simulink model "Active_Suspension_System"  (R2025b)
settings: Solver=ode45  StartTime=0.0  StopTime=10.0  RelTol=1e-3
undefined symbols (not defined in the file): cs, ct, Kd, Ki, Kp, ks, kt, ms, mus
libraries: slpidlib x1, simulink x1
settings Model: Creator=manikantagonugondla  LastModifiedBy=manikantagonugondla

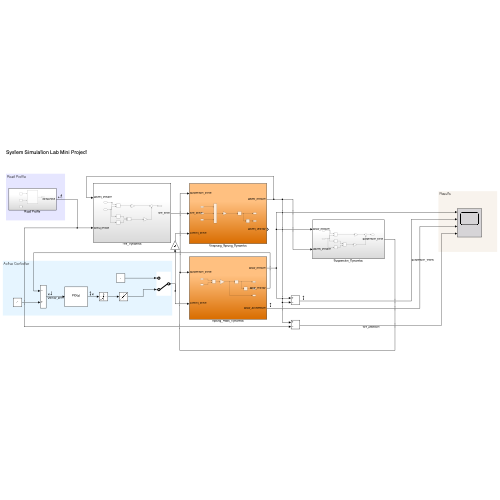
[thumbnail: Simulink's stored preview of the top-level diagram]
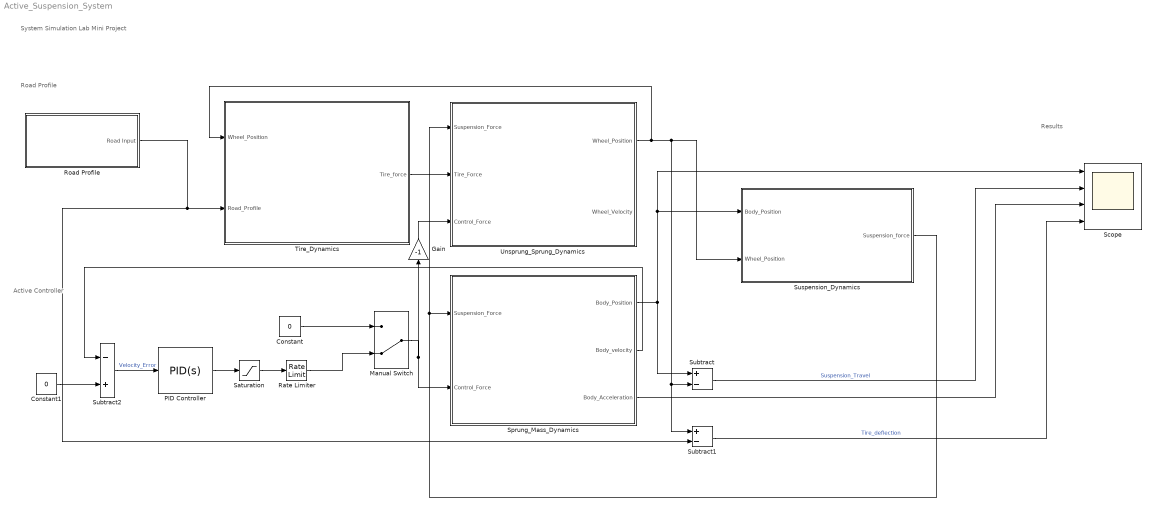
== system Active_Suspension_System ==
  note: Active Controller
  note: System Simulation Lab Mini Project
  note: Results
  note: Road Profile
  Constant : Constant  Value=0
  Constant1 : Constant  Value=0
  Gain : Gain  Gain=-1
  Manual Switch : ManualSwitch  CurrentSetting=0
  PID Controller : slpidlib/PID Controller  Controller=PID  Form=Parallel  TimeDomain=Continuous-time  UseExternalTs=off  SampleTime=-1  IntegratorMethod=Forward Euler  FilterMethod=Forward Euler  ControllerParametersSource=internal  P=Kp  I=Ki  UseKiTs=off  D=Kd  UseExternalDerivativeSource=off  N=50  UseFilter=on  TunerSelectOption=Transfer Function Based (PID Tuner App)  InitialConditionSource=internal  InitialConditionForIntegrator=0  InitialConditionForFilter=0  DifferentiatorICPrevScaledInput=0  ExternalReset=none  TrackingMode=off  Kt=1  LimitOutput=off  SatLimitsSource=internal  UpperSaturationLimit=inf  LowerSaturationLimit=-inf  LinearizeAsGain=on  AntiWindupMode=none  Kb=1  LimitIntegrator=off  UpperIntegratorSaturationLimit=inf  LowerIntegratorSaturationLimit=-inf  POutMin=[]  POutMax=[]  IOutMin=[]  IOutMax=[]  DOutMin=[]  DOutMax=[]  NOutMin=[]  NOutMax=[]  SumOutMin=[]  SumOutMax=[]  SaturationOutMin=[]  SaturationOutMax=[]  PParamMin=[]  PParamMax=[]  IParamMin=[]  IParamMax=[]  DParamMin=[]  DParamMax=[]  NParamMin=[]  NParamMax=[]  KbParamMin=[]  KbParamMax=[]  KtParamMin=[]  KtParamMax=[]  KbOutMin=[]  KbOutMax=[]  KtOutMin=[]  KtOutMax=[]  IntegratorOutMin=[]  IntegratorOutMax=[]  FilterOutMin=[]  FilterOutMax=[]  SumI1OutMin=[]  SumI1OutMax=[]  SumI2OutMin=[]  SumI2OutMax=[]  SumI3OutMin=[]  SumI3OutMax=[]  SumI4OutMin=[]  SumI4OutMax=[]  SumDOutMin=[]  SumDOutMax=[]  DifferentiatorOutMin=[]  DifferentiatorOutMax=[]  FilterDiffOutCoefMin=[]  FilterDiffOutCoefMax=[]  ReciprocalOutMin=[]  ReciprocalOutMax=[]  SumDenOutMin=[]  SumDenOutMax=[]  SumNumOutMin=[]  SumNumOutMax=[]  DivideOutMin=[]  DivideOutMax=[]  UdiffTsProdOutMin=[]  UdiffTsProdOutMax=[]  NTsProdOutMin=[]  NTsProdOutMax=[]  UintegralTsProdOutMin=[]  UintegralTsProdOutMax=[]  UngainTsProdOutMin=[]  UngainTsProdOutMax=[]  ClampingZeroOutDataTypeStr=Inherit: Inherit via back propagation  ClampingZeroOutMin=[]  ClampingZeroOutMax=[]  FilterDenConstantOutDataTypeStr=Inherit: Inherit via back propagation  FilterDenConstantOutMin=[]  FilterDenConstantOutMax=[]  PCopyOutDataTypeStr=Inherit: Inherit via back propagation  PCopyOutMin=[]  PCopyOutMax=[]  NCopyOutDataTypeStr=Inherit: Inherit via back propagation  NCopyOutMin=[]  NCopyOutMax=[]  IntegratorContinuousStateAttributes=''  IntegratorStateMustResolveToSignalObject=off  IntegratorRTWStateStorageClass=Auto  FilterContinuousStateAttributes=''  FilterStateMustResolveToSignalObject=off  FilterRTWStateStorageClass=Auto  ParallelPVariant=InternalParameters  IdealPVariant=Disabled  IVariant=InternalParameters  DVariant=InternalParameters  IntegratorVariant=Continuous  SatVariant=Disabled  AWVariant=Passthrough  PCopyVariant=Disabled  TRVariant=Disabled  FdbkBlocksVariant=Forward  IdealPFdbkVariant=Disabled  SatFdbkVariant=Disabled  DerivativeFilterVariant=ContFilter  NVariant=InternalParameters  NCopyVariant=Disabled  FilterICVariant=InternalICsFilter  IntegratorICVariant=InternalICs  ExternalResetVariant=Disabled  TRSumVariant=Passthrough  SumFdbkVariant=Disabled  SumVariant=Sum_PID  TsampFilterVariant=InternalTs  TsampNgainVariant=Passthrough  TsampIntegralVariant=Disabled_SignalSpec  ExternalSaturationOutDataTypeStr=Inherit: Same as second input  DerivativeSourceVariant=ErrorSignal  PreIntVariant=InternalPreInt
  Rate Limiter : RateLimiter  RisingSlewLimit=50000  FallingSlewLimit=-50000  SampleTimeMode=inherited
  Road Profile : Subsystem
  Saturation : Saturate  UpperLimit=5000  LowerLimit=-5000
  Scope : Scope  NumInputPorts=4
      settings: ActiveDisplayYMinimum=-0.0071336327558244837  ActiveDisplayYMaximum=0.064202694802420371
  Sprung_Mass_Dynamics : Subsystem
  Subtract : Sum  Inputs=+-
  Subtract1 : Sum  Inputs=+-
  Subtract2 : Sum  Inputs=-+
  Suspension_Dynamics : Subsystem
  Tire_Dynamics : Subsystem
  Unsprung_Sprung_Dynamics : Subsystem
  wires:
  Road Profile/1(Road Input) -> Subtract1/2, Tire_Dynamics/2(Road_Profile)
  Unsprung_Sprung_Dynamics/1(Wheel_Position) -> Subtract1/1, Subtract/2, Suspension_Dynamics/2(Wheel_Position), Tire_Dynamics/1(Wheel_Position)
  Tire_Dynamics/1(Tire_force) -> Unsprung_Sprung_Dynamics/2(Tire_Force)
  Sprung_Mass_Dynamics/1(Body_Position) -> Scope/1, Suspension_Dynamics/1(Body_Position), Subtract/1
  Suspension_Dynamics/1(Suspension_force) -> Sprung_Mass_Dynamics/1(Suspension_Force), Unsprung_Sprung_Dynamics/1(Suspension_Force)
  PID Controller/1 -> Saturation/1
  Sprung_Mass_Dynamics/3(Body_Acceleration) -> Scope/3
  Subtract/1 -> Scope/2  "Suspension_Travel"
  Subtract1/1 -> Scope/4  "Tire_deflection"
  Sprung_Mass_Dynamics/2(Body_velocity) -> Subtract2/1
  Constant1/1 -> Subtract2/2
  Subtract2/1 -> PID Controller/1  "Velocity_Error"
  Saturation/1 -> Rate Limiter/1
  Rate Limiter/1 -> Manual Switch/2
  Constant/1 -> Manual Switch/1
  Manual Switch/1 -> Sprung_Mass_Dynamics/2(Control_Force), Gain/1
  Gain/1 -> Unsprung_Sprung_Dynamics/3(Control_Force)

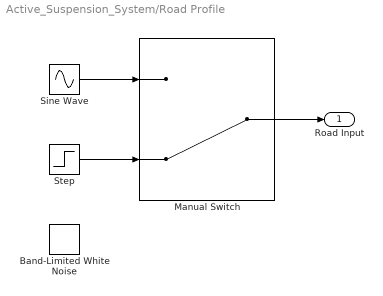
== system Active_Suspension_System/Road Profile ==
  Band-Limited White Noise : simulink/Sources/Band-Limited White Noise  Cov=[0.001]  Ts=0.01  seed=[23341]
  Manual Switch : ManualSwitch  CurrentSetting=0
  Sine Wave : Sin  Amplitude=0.03  Frequency=2*pi  SampleTime=0
  Step : Step  After=0.05  SampleTime=0
  Road Input : Outport
  wires:
  Sine Wave/1 -> Manual Switch/1
  Manual Switch/1 -> Road Input/1
  Step/1 -> Manual Switch/2

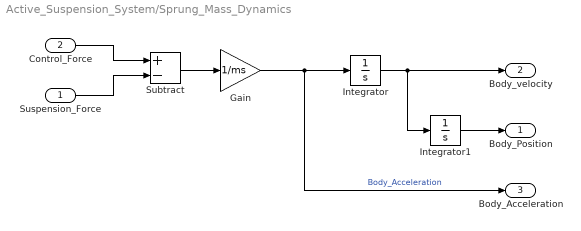
== system Active_Suspension_System/Sprung_Mass_Dynamics ==
  Suspension_Force : Inport
  Control_Force : Inport  Port=2
  Gain : Gain  Gain=1/ms
  Integrator : Integrator
  Integrator1 : Integrator
  Subtract : Sum  Inputs=+-
  Body_Position : Outport
  Body_velocity : Outport  Port=2
  Body_Acceleration : Outport  Port=3
  wires:
  Control_Force/1 -> Subtract/1
  Suspension_Force/1 -> Subtract/2
  Subtract/1 -> Gain/1
  Gain/1 -> Body_Acceleration/1, Integrator/1  "Body_Acceleration"
  Integrator/1 -> Integrator1/1, Body_velocity/1
  Integrator1/1 -> Body_Position/1

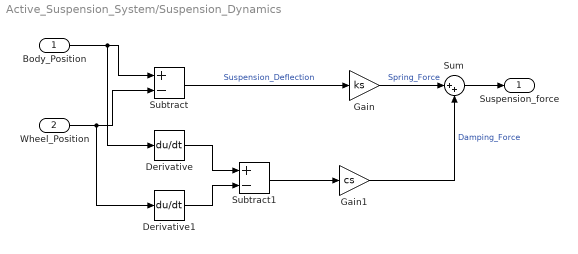
== system Active_Suspension_System/Suspension_Dynamics ==
  Body_Position : Inport
  Wheel_Position : Inport  Port=2
  Derivative : Derivative
  Derivative1 : Derivative
  Gain : Gain  Gain=ks
  Gain1 : Gain  Gain=cs
  Subtract : Sum  Inputs=+-
  Subtract1 : Sum  Inputs=+-
  Sum : Sum  Inputs=|++
  Suspension_force : Outport
  wires:
  Body_Position/1 -> Derivative/1, Subtract/1
  Wheel_Position/1 -> Derivative1/1, Subtract/2
  Subtract/1 -> Gain/1  "Suspension_Deflection"
  Derivative/1 -> Subtract1/1
  Derivative1/1 -> Subtract1/2
  Gain/1 -> Sum/1  "Spring_Force"
  Subtract1/1 -> Gain1/1
  Gain1/1 -> Sum/2  "Damping_Force"
  Sum/1 -> Suspension_force/1

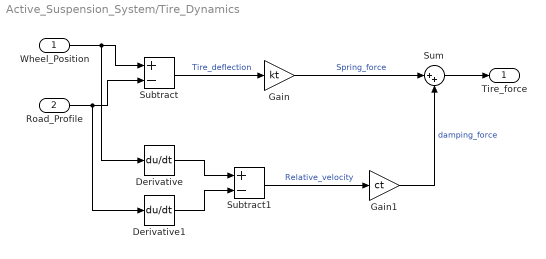
== system Active_Suspension_System/Tire_Dynamics ==
  Wheel_Position : Inport
  Road_Profile : Inport  Port=2
  Derivative : Derivative
  Derivative1 : Derivative
  Gain : Gain  Gain=kt
  Gain1 : Gain  Gain=ct
  Subtract : Sum  Inputs=+-
  Subtract1 : Sum  Inputs=+-
  Sum : Sum  Inputs=|++
  Tire_force : Outport
  wires:
  Wheel_Position/1 -> Derivative/1, Subtract/1
  Road_Profile/1 -> Derivative1/1, Subtract/2
  Subtract/1 -> Gain/1  "Tire_deflection"
  Gain/1 -> Sum/1  "Spring_force"
  Derivative/1 -> Subtract1/1
  Derivative1/1 -> Subtract1/2
  Subtract1/1 -> Gain1/1  "Relative_velocity"
  Gain1/1 -> Sum/2  "damping_force"
  Sum/1 -> Tire_force/1

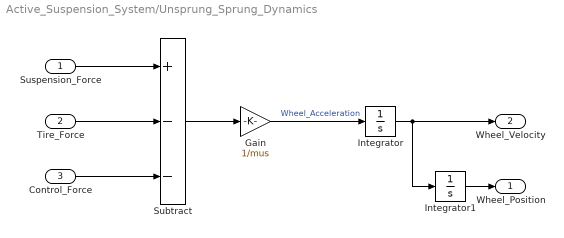
== system Active_Suspension_System/Unsprung_Sprung_Dynamics ==
  Suspension_Force : Inport
  Tire_Force : Inport  Port=2
  Control_Force : Inport  Port=3
  Gain : Gain  Gain=1/mus
  Integrator : Integrator
  Integrator1 : Integrator
  Subtract : Sum  Inputs=+--
  Wheel_Position : Outport
  Wheel_Velocity : Outport  Port=2
  wires:
  Suspension_Force/1 -> Subtract/1
  Tire_Force/1 -> Subtract/2
  Control_Force/1 -> Subtract/3
  Subtract/1 -> Gain/1
  Gain/1 -> Integrator/1  "Wheel_Acceleration"
  Integrator/1 -> Integrator1/1, Wheel_Velocity/1
  Integrator1/1 -> Wheel_Position/1
